simulink model "Project"  (R2021b)
settings: Solver=VariableStepAuto  StartTime=0.0  StopTime=4.0  RelTol=1e-3
values from neighbouring files (symbols this model uses):
  A = [0 1 0 0 ... (first row only)    [Inverted_pendulum.m]
  B = [0; 0.976; 0; -1.463;]    [Inverted_pendulum.m]
  C = eye(4,4)    [Inverted_pendulum.m]
  D = zeros(4,1)    [Inverted_pendulum.m]
  K = place(A,B,p)    [Inverted_pendulum.m]
  N = K*Nx+Nu    [Inverted_pendulum.m]
settings Model: Creator=merlis  LastModifiedBy=Merlis
settings SolverCC: AlgebraicLoopSolver=TrustRegion
settings DebuggingCC: SFMachineParentedDataDiag=warning

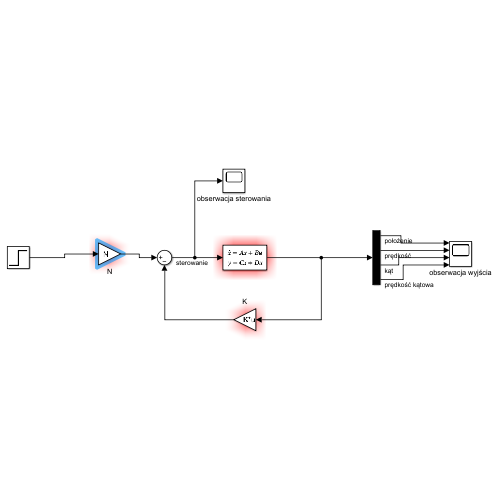
[thumbnail: Simulink's stored preview of the top-level diagram]
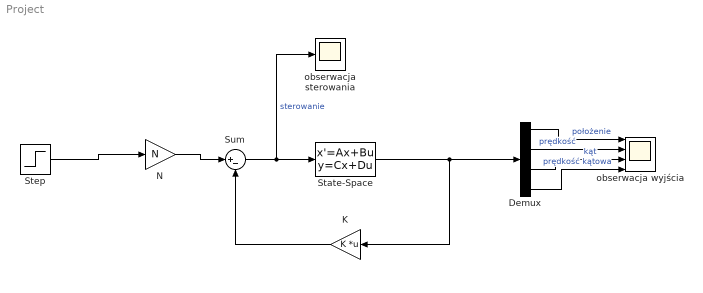
== system Project ==
  Demux : Demux
  K : Gain  Gain=K  Multiplication=Matrix(K*u)
  N : Gain  Gain=N
  State-Space : StateSpace  A=A  B=B  C=C  D=D  InitialCondition=[0; 0;0.15;0]
  Step : Step  Time=0  SampleTime=0
  Sum : Sum  Inputs=|+-
  obserwacja sterowania : Scope
  obserwacja wyjścia : Scope  NumInputPorts=4
  wires:
  N/1 -> Sum/1
  Step/1 -> N/1
  Sum/1 -> obserwacja sterowania/1, State-Space/1  "sterowanie"
  State-Space/1 -> K/1, Demux/1
  K/1 -> Sum/2
  Demux/1 -> obserwacja wyjścia/1  "położenie"
  Demux/2 -> obserwacja wyjścia/2  "prędkość"
  Demux/3 -> obserwacja wyjścia/3  "kąt"
  Demux/4 -> obserwacja wyjścia/4  "prędkość kątowa"
